simulink model "TST_PIntkVUs_DD"  (R2016b)
settings: Solver=FixedStepDiscrete  StartTime=0.0  StopTime=simTime  FixedStep=sampleTime  RelTol=1e-3
values from neighbouring files (symbols this model uses):
  testCase = 1    [initTST_PIntkVUs_DD_001.m]    (also in initTST_PIntkVUs_DD_002.m = 2; initTST_PIntkVUs_DD_003.m = 3; initTST_PIntkVUs_DD_004.m = 4; initTST_PIntkVUs_DD_005.m = 5)
libraries: UnitTest_Lib x98, simulink x8
(part 1 of 3)
settings Model: Creator=liangyunbo  LastModifiedBy=liangyunbo
settings DebuggingCC: SignalRangeChecking=error

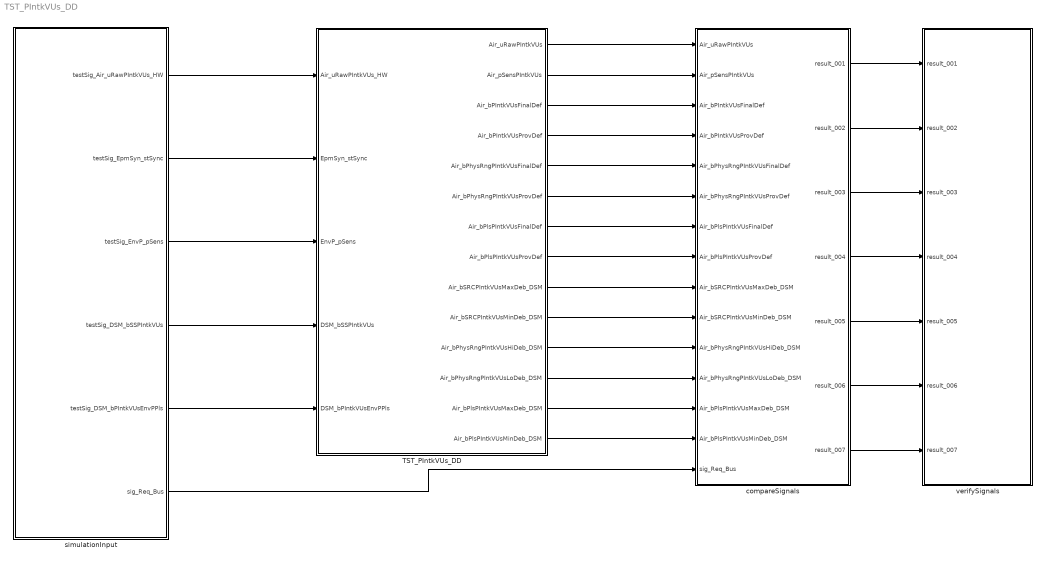
== system TST_PIntkVUs_DD ==
  TST_PIntkVUs_DD : Subsystem
  compareSignals : Subsystem
  simulationInput : Subsystem
  verifySignals : Subsystem
  wires:
  simulationInput/1(testSig_Air_uRawPIntkVUs_HW) -> TST_PIntkVUs_DD/1(Air_uRawPIntkVUs_HW)
  simulationInput/2(testSig_EpmSyn_stSync) -> TST_PIntkVUs_DD/2(EpmSyn_stSync)
  simulationInput/3(testSig_EnvP_pSens) -> TST_PIntkVUs_DD/3(EnvP_pSens)
  simulationInput/4(testSig_DSM_bSSPIntkVUs) -> TST_PIntkVUs_DD/4(DSM_bSSPIntkVUs)
  simulationInput/5(testSig_DSM_bPIntkVUsEnvPPls) -> TST_PIntkVUs_DD/5(DSM_bPIntkVUsEnvPPls)
  TST_PIntkVUs_DD/1(Air_uRawPIntkVUs) -> compareSignals/1(Air_uRawPIntkVUs)
  TST_PIntkVUs_DD/2(Air_pSensPIntkVUs) -> compareSignals/2(Air_pSensPIntkVUs)
  TST_PIntkVUs_DD/3(Air_bPIntkVUsFinalDef) -> compareSignals/3(Air_bPIntkVUsFinalDef)
  TST_PIntkVUs_DD/4(Air_bPIntkVUsProvDef) -> compareSignals/4(Air_bPIntkVUsProvDef)
  TST_PIntkVUs_DD/5(Air_bPhysRngPIntkVUsFinalDef) -> compareSignals/5(Air_bPhysRngPIntkVUsFinalDef)
  TST_PIntkVUs_DD/6(Air_bPhysRngPIntkVUsProvDef) -> compareSignals/6(Air_bPhysRngPIntkVUsProvDef)
  TST_PIntkVUs_DD/7(Air_bPlsPIntkVUsFinalDef) -> compareSignals/7(Air_bPlsPIntkVUsFinalDef)
  TST_PIntkVUs_DD/8(Air_bPlsPIntkVUsProvDef) -> compareSignals/8(Air_bPlsPIntkVUsProvDef)
  TST_PIntkVUs_DD/9(Air_bSRCPIntkVUsMaxDeb_DSM) -> compareSignals/9(Air_bSRCPIntkVUsMaxDeb_DSM)
  TST_PIntkVUs_DD/10(Air_bSRCPIntkVUsMinDeb_DSM) -> compareSignals/10(Air_bSRCPIntkVUsMinDeb_DSM)
  TST_PIntkVUs_DD/11(Air_bPhysRngPIntkVUsHiDeb_DSM) -> compareSignals/11(Air_bPhysRngPIntkVUsHiDeb_DSM)
  TST_PIntkVUs_DD/12(Air_bPhysRngPIntkVUsLoDeb_DSM) -> compareSignals/12(Air_bPhysRngPIntkVUsLoDeb_DSM)
  TST_PIntkVUs_DD/13(Air_bPlsPIntkVUsMaxDeb_DSM) -> compareSignals/13(Air_bPlsPIntkVUsMaxDeb_DSM)
  TST_PIntkVUs_DD/14(Air_bPlsPIntkVUsMinDeb_DSM) -> compareSignals/14(Air_bPlsPIntkVUsMinDeb_DSM)
  simulationInput/6(sig_Req_Bus) -> compareSignals/15(sig_Req_Bus)
  compareSignals/1(result_001) -> verifySignals/1(result_001)
  compareSignals/2(result_002) -> verifySignals/2(result_002)
  compareSignals/3(result_003) -> verifySignals/3(result_003)
  compareSignals/4(result_004) -> verifySignals/4(result_004)
  compareSignals/5(result_005) -> verifySignals/5(result_005)
  compareSignals/6(result_006) -> verifySignals/6(result_006)
  compareSignals/7(result_007) -> verifySignals/7(result_007)

== system TST_PIntkVUs_DD/TST_PIntkVUs_DD ==
  Air_uRawPIntkVUs_HW : Inport
  EpmSyn_stSync : Inport  Port=2
  EnvP_pSens : Inport  Port=3
  DSM_bSSPIntkVUs : Inport  Port=4
  DSM_bPIntkVUsEnvPPls : Inport  Port=5
  Function_Call : simulink/Ports & Subsystems/Function-Call Generator  sample_time=sampleTime  numberOfIterations=1
  PIntkVUs_DD : ModelReference  ModelNameDialog=PIntkVUs_DD  SimulationMode=Normal  ModelReferenceVersion=1.45  TriggerPortName=function  TriggerPortTriggerType=function-call  TriggerPortStatesWhenEnabling=held
  Air_uRawPIntkVUs : Outport
  Air_pSensPIntkVUs : Outport  Port=2
  Air_bPIntkVUsFinalDef : Outport  Port=3
  Air_bPIntkVUsProvDef : Outport  Port=4
  Air_bPhysRngPIntkVUsFinalDef : Outport  Port=5
  Air_bPhysRngPIntkVUsProvDef : Outport  Port=6
  Air_bPlsPIntkVUsFinalDef : Outport  Port=7
  Air_bPlsPIntkVUsProvDef : Outport  Port=8
  Air_bSRCPIntkVUsMaxDeb_DSM : Outport  Port=9
  Air_bSRCPIntkVUsMinDeb_DSM : Outport  Port=10
  Air_bPhysRngPIntkVUsHiDeb_DSM : Outport  Port=11
  Air_bPhysRngPIntkVUsLoDeb_DSM : Outport  Port=12
  Air_bPlsPIntkVUsMaxDeb_DSM : Outport  Port=13
  Air_bPlsPIntkVUsMinDeb_DSM : Outport  Port=14
  wires:
  Function_Call/1 -> PIntkVUs_DD/Trigger
  Air_uRawPIntkVUs_HW/1 -> PIntkVUs_DD/1
  EpmSyn_stSync/1 -> PIntkVUs_DD/2
  EnvP_pSens/1 -> PIntkVUs_DD/3
  DSM_bSSPIntkVUs/1 -> PIntkVUs_DD/4
  DSM_bPIntkVUsEnvPPls/1 -> PIntkVUs_DD/5
  PIntkVUs_DD/1 -> Air_uRawPIntkVUs/1
  PIntkVUs_DD/2 -> Air_pSensPIntkVUs/1
  PIntkVUs_DD/3 -> Air_bPIntkVUsFinalDef/1
  PIntkVUs_DD/4 -> Air_bPIntkVUsProvDef/1
  PIntkVUs_DD/5 -> Air_bPhysRngPIntkVUsFinalDef/1
  PIntkVUs_DD/6 -> Air_bPhysRngPIntkVUsProvDef/1
  PIntkVUs_DD/7 -> Air_bPlsPIntkVUsFinalDef/1
  PIntkVUs_DD/8 -> Air_bPlsPIntkVUsProvDef/1
  PIntkVUs_DD/9 -> Air_bSRCPIntkVUsMaxDeb_DSM/1
  PIntkVUs_DD/10 -> Air_bSRCPIntkVUsMinDeb_DSM/1
  PIntkVUs_DD/11 -> Air_bPhysRngPIntkVUsHiDeb_DSM/1
  PIntkVUs_DD/12 -> Air_bPhysRngPIntkVUsLoDeb_DSM/1
  PIntkVUs_DD/13 -> Air_bPlsPIntkVUsMaxDeb_DSM/1
  PIntkVUs_DD/14 -> Air_bPlsPIntkVUsMinDeb_DSM/1

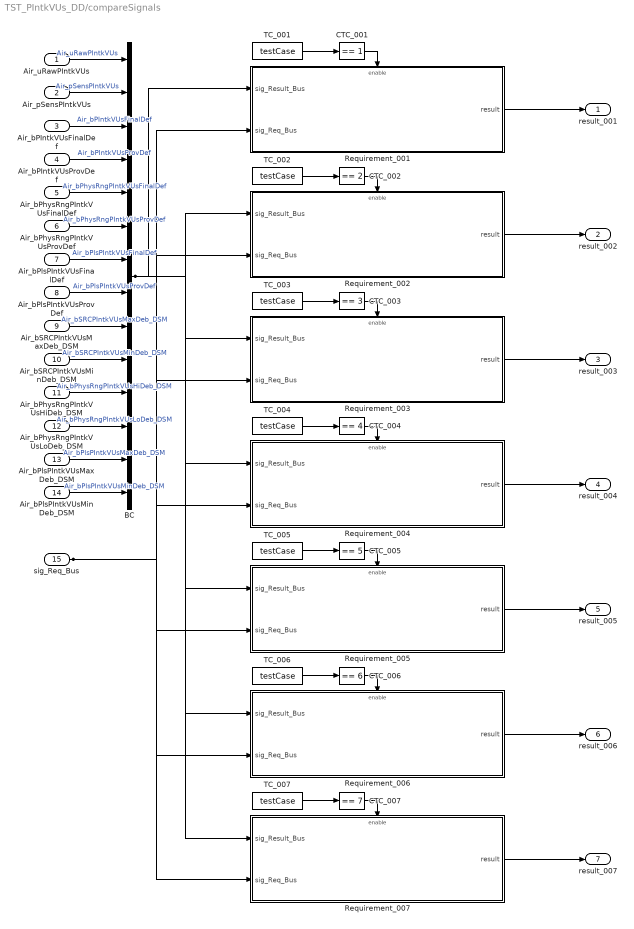
== system TST_PIntkVUs_DD/compareSignals ==
  Air_uRawPIntkVUs : Inport
  Air_pSensPIntkVUs : Inport  Port=2
  Air_bPIntkVUsFinalDef : Inport  Port=3
  Air_bPIntkVUsProvDef : Inport  Port=4
  Air_bPhysRngPIntkVUsFinalDef : Inport  Port=5
  Air_bPhysRngPIntkVUsProvDef : Inport  Port=6
  Air_bPlsPIntkVUsFinalDef : Inport  Port=7
  Air_bPlsPIntkVUsProvDef : Inport  Port=8
  Air_bSRCPIntkVUsMaxDeb_DSM : Inport  Port=9
  Air_bSRCPIntkVUsMinDeb_DSM : Inport  Port=10
  Air_bPhysRngPIntkVUsHiDeb_DSM : Inport  Port=11
  Air_bPhysRngPIntkVUsLoDeb_DSM : Inport  Port=12
  Air_bPlsPIntkVUsMaxDeb_DSM : Inport  Port=13
  Air_bPlsPIntkVUsMinDeb_DSM : Inport  Port=14
  sig_Req_Bus : Inport  Port=15
  BC : BusCreator  Inputs=14
  CTC_001 : simulink/Logic and Bit Operations/Compare To Constant  relop===  const=1  OutDataTypeStr=boolean
  CTC_002 : simulink/Logic and Bit Operations/Compare To Constant  relop===  const=2  OutDataTypeStr=boolean
  CTC_003 : simulink/Logic and Bit Operations/Compare To Constant  relop===  const=3  OutDataTypeStr=boolean
  CTC_004 : simulink/Logic and Bit Operations/Compare To Constant  relop===  const=4  OutDataTypeStr=boolean
  CTC_005 : simulink/Logic and Bit Operations/Compare To Constant  relop===  const=5  OutDataTypeStr=boolean
  CTC_006 : simulink/Logic and Bit Operations/Compare To Constant  relop===  const=6  OutDataTypeStr=boolean
  CTC_007 : simulink/Logic and Bit Operations/Compare To Constant  relop===  const=7  OutDataTypeStr=boolean
  Requirement_001 : Subsystem
  Requirement_002 : Subsystem
  Requirement_003 : Subsystem
  Requirement_004 : Subsystem
  Requirement_005 : Subsystem
  Requirement_006 : Subsystem
  Requirement_007 : Subsystem
  TC_001 : Constant  Value=testCase
  TC_002 : Constant  Value=testCase
  TC_003 : Constant  Value=testCase
  TC_004 : Constant  Value=testCase
  TC_005 : Constant  Value=testCase
  TC_006 : Constant  Value=testCase
  TC_007 : Constant  Value=testCase
  result_001 : Outport
  result_002 : Outport  Port=2
  result_003 : Outport  Port=3
  result_004 : Outport  Port=4
  result_005 : Outport  Port=5
  result_006 : Outport  Port=6
  result_007 : Outport  Port=7
  wires:
  Air_uRawPIntkVUs/1 -> BC/1  "Air_uRawPIntkVUs"
  Air_pSensPIntkVUs/1 -> BC/2  "Air_pSensPIntkVUs"
  Air_bPIntkVUsFinalDef/1 -> BC/3  "Air_bPIntkVUsFinalDef"
  Air_bPIntkVUsProvDef/1 -> BC/4  "Air_bPIntkVUsProvDef"
  Air_bPhysRngPIntkVUsFinalDef/1 -> BC/5  "Air_bPhysRngPIntkVUsFinalDef"
  Air_bPhysRngPIntkVUsProvDef/1 -> BC/6  "Air_bPhysRngPIntkVUsProvDef"
  Air_bPlsPIntkVUsFinalDef/1 -> BC/7  "Air_bPlsPIntkVUsFinalDef"
  Air_bPlsPIntkVUsProvDef/1 -> BC/8  "Air_bPlsPIntkVUsProvDef"
  Air_bSRCPIntkVUsMaxDeb_DSM/1 -> BC/9  "Air_bSRCPIntkVUsMaxDeb_DSM"
  Air_bSRCPIntkVUsMinDeb_DSM/1 -> BC/10  "Air_bSRCPIntkVUsMinDeb_DSM"
  Air_bPhysRngPIntkVUsHiDeb_DSM/1 -> BC/11  "Air_bPhysRngPIntkVUsHiDeb_DSM"
  Air_bPhysRngPIntkVUsLoDeb_DSM/1 -> BC/12  "Air_bPhysRngPIntkVUsLoDeb_DSM"
  Air_bPlsPIntkVUsMaxDeb_DSM/1 -> BC/13  "Air_bPlsPIntkVUsMaxDeb_DSM"
  Air_bPlsPIntkVUsMinDeb_DSM/1 -> BC/14  "Air_bPlsPIntkVUsMinDeb_DSM"
  TC_001/1 -> CTC_001/1
  CTC_001/1 -> Requirement_001/Enable
  sig_Req_Bus/1 -> Requirement_001/2(sig_Req_Bus), Requirement_002/2(sig_Req_Bus), Requirement_003/2(sig_Req_Bus), Requirement_004/2(sig_Req_Bus), Requirement_005/2(sig_Req_Bus), Requirement_006/2(sig_Req_Bus), Requirement_007/2(sig_Req_Bus)
  BC/1 -> Requirement_001/1(sig_Result_Bus), Requirement_002/1(sig_Result_Bus), Requirement_003/1(sig_Result_Bus), Requirement_004/1(sig_Result_Bus), Requirement_005/1(sig_Result_Bus), Requirement_006/1(sig_Result_Bus), Requirement_007/1(sig_Result_Bus)
  Requirement_001/1(result) -> result_001/1
  TC_002/1 -> CTC_002/1
  CTC_002/1 -> Requirement_002/Enable
  Requirement_002/1(result) -> result_002/1
  TC_003/1 -> CTC_003/1
  CTC_003/1 -> Requirement_003/Enable
  Requirement_003/1(result) -> result_003/1
  TC_004/1 -> CTC_004/1
  CTC_004/1 -> Requirement_004/Enable
  Requirement_004/1(result) -> result_004/1
  TC_005/1 -> CTC_005/1
  CTC_005/1 -> Requirement_005/Enable
  Requirement_005/1(result) -> result_005/1
  TC_006/1 -> CTC_006/1
  CTC_006/1 -> Requirement_006/Enable
  Requirement_006/1(result) -> result_006/1
  TC_007/1 -> CTC_007/1
  CTC_007/1 -> Requirement_007/Enable
  Requirement_007/1(result) -> result_007/1

== system TST_PIntkVUs_DD/simulationInput ==
  BS : BusSelector  OutputSignals=testSig_Air_uRawPIntkVUs_HW,testSig_EpmSyn_stSync,testSig_EnvP_pSens,testSig_DSM_bSSPIntkVUs,testSig_DSM_bPIntkVUsEnvPPls
  MPSw : MultiPortSwitch  Inputs=7  SaturateOnIntegerOverflow=on  InputSameDT=on
  TestCase : Constant  Value=testCase
  testSignals_R001 : Subsystem
  testSignals_R002 : Subsystem
  testSignals_R003 : Subsystem
  testSignals_R004 : Subsystem
  testSignals_R005 : Subsystem
  testSignals_R006 : Subsystem
  testSignals_R007 : Subsystem
  testSig_Air_uRawPIntkVUs_HW : Outport
  testSig_EpmSyn_stSync : Outport  Port=2
  testSig_EnvP_pSens : Outport  Port=3
  testSig_DSM_bSSPIntkVUs : Outport  Port=4
  testSig_DSM_bPIntkVUsEnvPPls : Outport  Port=5
  sig_Req_Bus : Outport  Port=6
  wires:
  BS/1 -> testSig_Air_uRawPIntkVUs_HW/1  "<testSig_Air_uRawPIntkVUs_HW>"
  BS/2 -> testSig_EpmSyn_stSync/1  "<testSig_EpmSyn_stSync>"
  BS/3 -> testSig_EnvP_pSens/1  "<testSig_EnvP_pSens>"
  BS/4 -> testSig_DSM_bSSPIntkVUs/1  "<testSig_DSM_bSSPIntkVUs>"
  BS/5 -> testSig_DSM_bPIntkVUsEnvPPls/1  "<testSig_DSM_bPIntkVUsEnvPPls>"
  MPSw/1 -> BS/1, sig_Req_Bus/1
  TestCase/1 -> MPSw/1
  testSignals_R001/1(testSignals) -> MPSw/2
  testSignals_R002/1(testSignals) -> MPSw/3
  testSignals_R003/1(testSignals) -> MPSw/4
  testSignals_R004/1(testSignals) -> MPSw/5
  testSignals_R005/1(testSignals) -> MPSw/6
  testSignals_R006/1(testSignals) -> MPSw/7
  testSignals_R007/1(testSignals) -> MPSw/8

== system TST_PIntkVUs_DD/verifySignals ==
  result_001 : Inport
  result_002 : Inport  Port=2
  result_003 : Inport  Port=3
  result_004 : Inport  Port=4
  result_005 : Inport  Port=5
  result_006 : Inport  Port=6
  result_007 : Inport  Port=7
  Assertion_001 : Assertion  Enabled=off
  Assertion_002 : Assertion  Enabled=off
  Assertion_003 : Assertion  Enabled=off
  Assertion_004 : Assertion  Enabled=off
  Assertion_005 : Assertion  Enabled=off
  Assertion_006 : Assertion  Enabled=off
  Assertion_007 : Assertion  Enabled=off
  wires:
  result_001/1 -> Assertion_001/1
  result_002/1 -> Assertion_002/1
  result_003/1 -> Assertion_003/1
  result_004/1 -> Assertion_004/1
  result_005/1 -> Assertion_005/1
  result_006/1 -> Assertion_006/1
  result_007/1 -> Assertion_007/1

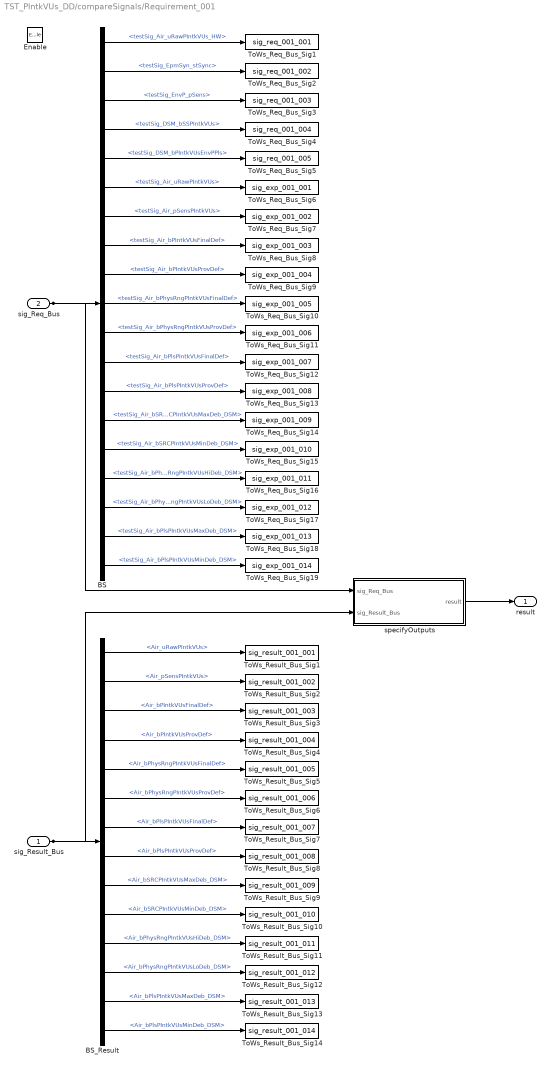
== system TST_PIntkVUs_DD/compareSignals/Requirement_001 ==
  sig_Result_Bus : Inport
  sig_Req_Bus : Inport  Port=2
  Enable : EnablePort
  BS : BusSelector  OutputSignals=testSig_Air_uRawPIntkVUs_HW,testSig_EpmSyn_stSync,testSig_EnvP_pSens,testSig_DSM_bSSPIntkVUs,testSig_DSM_bPIntkVUsEnvPPls,testSig_Air_uRawPIntkVUs,testSig_Air_pSensPIntkVUs,testSig_Air_bPIntkVUsFinalDef,testSig_Air_bPIntkVUsProvDef,testSig_Air_bPhysRngPIntkVUsFinalDef,testSig_Air_bPhysRngPIntkVUsProvDef,testSig_Air_bPlsPIntkVUsFinalDef,testSig_Air_bPlsPIntkVUsProvDef,testSig_Air_bSRCPIntkVUsMaxDeb_DSM,testSig_Air_bSRCPIntkVUsMinDeb_DSM,testSig_Air_bPhysRngPIntkVUsHiDeb_DSM,testSig_Air_bPhysRngPIntkVUsLoDeb_DSM,testSig_Air_bPlsPIntkVUsMaxDeb_DSM,testSig_Air_bPlsPIntkVUsMinDeb_DSM
  BS_Result : BusSelector  OutputSignals=Air_uRawPIntkVUs,Air_pSensPIntkVUs,Air_bPIntkVUsFinalDef,Air_bPIntkVUsProvDef,Air_bPhysRngPIntkVUsFinalDef,Air_bPhysRngPIntkVUsProvDef,Air_bPlsPIntkVUsFinalDef,Air_bPlsPIntkVUsProvDef,Air_bSRCPIntkVUsMaxDeb_DSM,Air_bSRCPIntkVUsMinDeb_DSM,Air_bPhysRngPIntkVUsHiDeb_DSM,Air_bPhysRngPIntkVUsLoDeb_DSM,Air_bPlsPIntkVUsMaxDeb_DSM,Air_bPlsPIntkVUsMinDeb_DSM
  ToWs_Req_Bus_Sig1 : ToWorkspace  VariableName=sig_req_001_001  SaveFormat=Structure With Time
  ToWs_Req_Bus_Sig10 : ToWorkspace  VariableName=sig_exp_001_005  SaveFormat=Structure With Time
  ToWs_Req_Bus_Sig11 : ToWorkspace  VariableName=sig_exp_001_006  SaveFormat=Structure With Time
  ToWs_Req_Bus_Sig12 : ToWorkspace  VariableName=sig_exp_001_007  SaveFormat=Structure With Time
  ToWs_Req_Bus_Sig13 : ToWorkspace  VariableName=sig_exp_001_008  SaveFormat=Structure With Time
  ToWs_Req_Bus_Sig14 : ToWorkspace  VariableName=sig_exp_001_009  SaveFormat=Structure With Time
  ToWs_Req_Bus_Sig15 : ToWorkspace  VariableName=sig_exp_001_010  SaveFormat=Structure With Time
  ToWs_Req_Bus_Sig16 : ToWorkspace  VariableName=sig_exp_001_011  SaveFormat=Structure With Time
  ToWs_Req_Bus_Sig17 : ToWorkspace  VariableName=sig_exp_001_012  SaveFormat=Structure With Time
  ToWs_Req_Bus_Sig18 : ToWorkspace  VariableName=sig_exp_001_013  SaveFormat=Structure With Time
  ToWs_Req_Bus_Sig19 : ToWorkspace  VariableName=sig_exp_001_014  SaveFormat=Structure With Time
  ToWs_Req_Bus_Sig2 : ToWorkspace  VariableName=sig_req_001_002  SaveFormat=Structure With Time
  ToWs_Req_Bus_Sig3 : ToWorkspace  VariableName=sig_req_001_003  SaveFormat=Structure With Time
  ToWs_Req_Bus_Sig4 : ToWorkspace  VariableName=sig_req_001_004  SaveFormat=Structure With Time
  ToWs_Req_Bus_Sig5 : ToWorkspace  VariableName=sig_req_001_005  SaveFormat=Structure With Time
  ToWs_Req_Bus_Sig6 : ToWorkspace  VariableName=sig_exp_001_001  SaveFormat=Structure With Time
  ToWs_Req_Bus_Sig7 : ToWorkspace  VariableName=sig_exp_001_002  SaveFormat=Structure With Time
  ToWs_Req_Bus_Sig8 : ToWorkspace  VariableName=sig_exp_001_003  SaveFormat=Structure With Time
  ToWs_Req_Bus_Sig9 : ToWorkspace  VariableName=sig_exp_001_004  SaveFormat=Structure With Time
  ToWs_Result_Bus_Sig1 : ToWorkspace  VariableName=sig_result_001_001  SaveFormat=Structure With Time
  ToWs_Result_Bus_Sig10 : ToWorkspace  VariableName=sig_result_001_010  SaveFormat=Structure With Time
  ToWs_Result_Bus_Sig11 : ToWorkspace  VariableName=sig_result_001_011  SaveFormat=Structure With Time
  ToWs_Result_Bus_Sig12 : ToWorkspace  VariableName=sig_result_001_012  SaveFormat=Structure With Time
  ToWs_Result_Bus_Sig13 : ToWorkspace  VariableName=sig_result_001_013  SaveFormat=Structure With Time
  ToWs_Result_Bus_Sig14 : ToWorkspace  VariableName=sig_result_001_014  SaveFormat=Structure With Time
  ToWs_Result_Bus_Sig2 : ToWorkspace  VariableName=sig_result_001_002  SaveFormat=Structure With Time
  ToWs_Result_Bus_Sig3 : ToWorkspace  VariableName=sig_result_001_003  SaveFormat=Structure With Time
  ToWs_Result_Bus_Sig4 : ToWorkspace  VariableName=sig_result_001_004  SaveFormat=Structure With Time
  ToWs_Result_Bus_Sig5 : ToWorkspace  VariableName=sig_result_001_005  SaveFormat=Structure With Time
  ToWs_Result_Bus_Sig6 : ToWorkspace  VariableName=sig_result_001_006  SaveFormat=Structure With Time
  ToWs_Result_Bus_Sig7 : ToWorkspace  VariableName=sig_result_001_007  SaveFormat=Structure With Time
  ToWs_Result_Bus_Sig8 : ToWorkspace  VariableName=sig_result_001_008  SaveFormat=Structure With Time
  ToWs_Result_Bus_Sig9 : ToWorkspace  VariableName=sig_result_001_009  SaveFormat=Structure With Time
  specifyOutputs : Subsystem
  result : Outport
  wires:
  sig_Req_Bus/1 -> BS/1, specifyOutputs/1(sig_Req_Bus)
  BS/1 -> ToWs_Req_Bus_Sig1/1  "<testSig_Air_uRawPIntkVUs_HW>"
  BS/2 -> ToWs_Req_Bus_Sig2/1  "<testSig_EpmSyn_stSync>"
  BS/3 -> ToWs_Req_Bus_Sig3/1  "<testSig_EnvP_pSens>"
  BS/4 -> ToWs_Req_Bus_Sig4/1  "<testSig_DSM_bSSPIntkVUs>"
  BS/5 -> ToWs_Req_Bus_Sig5/1  "<testSig_DSM_bPIntkVUsEnvPPls>"
  BS/6 -> ToWs_Req_Bus_Sig6/1  "<testSig_Air_uRawPIntkVUs>"
  BS/7 -> ToWs_Req_Bus_Sig7/1  "<testSig_Air_pSensPIntkVUs>"
  BS/8 -> ToWs_Req_Bus_Sig8/1  "<testSig_Air_bPIntkVUsFinalDef>"
  BS/9 -> ToWs_Req_Bus_Sig9/1  "<testSig_Air_bPIntkVUsProvDef>"
  BS/10 -> ToWs_Req_Bus_Sig10/1  "<testSig_Air_bPhysRngPIntkVUsFinalDef>"
  BS/11 -> ToWs_Req_Bus_Sig11/1  "<testSig_Air_bPhysRngPIntkVUsProvDef>"
  BS/12 -> ToWs_Req_Bus_Sig12/1  "<testSig_Air_bPlsPIntkVUsFinalDef>"
  BS/13 -> ToWs_Req_Bus_Sig13/1  "<testSig_Air_bPlsPIntkVUsProvDef>"
  BS/14 -> ToWs_Req_Bus_Sig14/1  "<testSig_Air_bSRCPIntkVUsMaxDeb_DSM>"
  BS/15 -> ToWs_Req_Bus_Sig15/1  "<testSig_Air_bSRCPIntkVUsMinDeb_DSM>"
  BS/16 -> ToWs_Req_Bus_Sig16/1  "<testSig_Air_bPhysRngPIntkVUsHiDeb_DSM>"
  BS/17 -> ToWs_Req_Bus_Sig17/1  "<testSig_Air_bPhysRngPIntkVUsLoDeb_DSM>"
  BS/18 -> ToWs_Req_Bus_Sig18/1  "<testSig_Air_bPlsPIntkVUsMaxDeb_DSM>"
  BS/19 -> ToWs_Req_Bus_Sig19/1  "<testSig_Air_bPlsPIntkVUsMinDeb_DSM>"
  sig_Result_Bus/1 -> BS_Result/1, specifyOutputs/2(sig_Result_Bus)
  BS_Result/1 -> ToWs_Result_Bus_Sig1/1  "<Air_uRawPIntkVUs>"
  BS_Result/2 -> ToWs_Result_Bus_Sig2/1  "<Air_pSensPIntkVUs>"
  BS_Result/3 -> ToWs_Result_Bus_Sig3/1  "<Air_bPIntkVUsFinalDef>"
  BS_Result/4 -> ToWs_Result_Bus_Sig4/1  "<Air_bPIntkVUsProvDef>"
  BS_Result/5 -> ToWs_Result_Bus_Sig5/1  "<Air_bPhysRngPIntkVUsFinalDef>"
  BS_Result/6 -> ToWs_Result_Bus_Sig6/1  "<Air_bPhysRngPIntkVUsProvDef>"
  BS_Result/7 -> ToWs_Result_Bus_Sig7/1  "<Air_bPlsPIntkVUsFinalDef>"
  BS_Result/8 -> ToWs_Result_Bus_Sig8/1  "<Air_bPlsPIntkVUsProvDef>"
  BS_Result/9 -> ToWs_Result_Bus_Sig9/1  "<Air_bSRCPIntkVUsMaxDeb_DSM>"
  BS_Result/10 -> ToWs_Result_Bus_Sig10/1  "<Air_bSRCPIntkVUsMinDeb_DSM>"
  BS_Result/11 -> ToWs_Result_Bus_Sig11/1  "<Air_bPhysRngPIntkVUsHiDeb_DSM>"
  BS_Result/12 -> ToWs_Result_Bus_Sig12/1  "<Air_bPhysRngPIntkVUsLoDeb_DSM>"
  BS_Result/13 -> ToWs_Result_Bus_Sig13/1  "<Air_bPlsPIntkVUsMaxDeb_DSM>"
  BS_Result/14 -> ToWs_Result_Bus_Sig14/1  "<Air_bPlsPIntkVUsMinDeb_DSM>"
  specifyOutputs/1(result) -> result/1

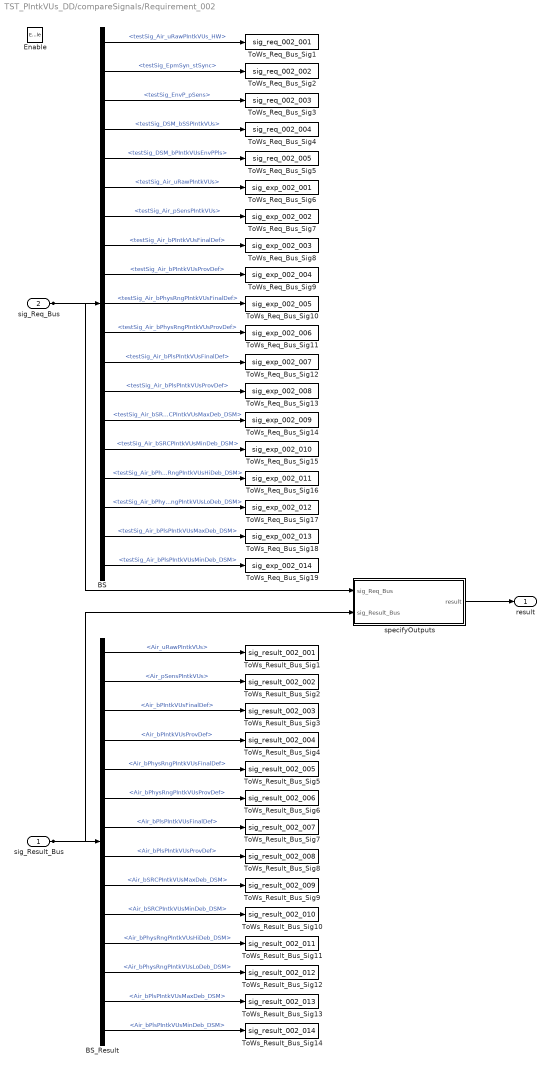
== system TST_PIntkVUs_DD/compareSignals/Requirement_002 ==
  sig_Result_Bus : Inport
  sig_Req_Bus : Inport  Port=2
  Enable : EnablePort
  BS : BusSelector  OutputSignals=testSig_Air_uRawPIntkVUs_HW,testSig_EpmSyn_stSync,testSig_EnvP_pSens,testSig_DSM_bSSPIntkVUs,testSig_DSM_bPIntkVUsEnvPPls,testSig_Air_uRawPIntkVUs,testSig_Air_pSensPIntkVUs,testSig_Air_bPIntkVUsFinalDef,testSig_Air_bPIntkVUsProvDef,testSig_Air_bPhysRngPIntkVUsFinalDef,testSig_Air_bPhysRngPIntkVUsProvDef,testSig_Air_bPlsPIntkVUsFinalDef,testSig_Air_bPlsPIntkVUsProvDef,testSig_Air_bSRCPIntkVUsMaxDeb_DSM,testSig_Air_bSRCPIntkVUsMinDeb_DSM,testSig_Air_bPhysRngPIntkVUsHiDeb_DSM,testSig_Air_bPhysRngPIntkVUsLoDeb_DSM,testSig_Air_bPlsPIntkVUsMaxDeb_DSM,testSig_Air_bPlsPIntkVUsMinDeb_DSM
  BS_Result : BusSelector  OutputSignals=Air_uRawPIntkVUs,Air_pSensPIntkVUs,Air_bPIntkVUsFinalDef,Air_bPIntkVUsProvDef,Air_bPhysRngPIntkVUsFinalDef,Air_bPhysRngPIntkVUsProvDef,Air_bPlsPIntkVUsFinalDef,Air_bPlsPIntkVUsProvDef,Air_bSRCPIntkVUsMaxDeb_DSM,Air_bSRCPIntkVUsMinDeb_DSM,Air_bPhysRngPIntkVUsHiDeb_DSM,Air_bPhysRngPIntkVUsLoDeb_DSM,Air_bPlsPIntkVUsMaxDeb_DSM,Air_bPlsPIntkVUsMinDeb_DSM
  ToWs_Req_Bus_Sig1 : ToWorkspace  VariableName=sig_req_002_001  SaveFormat=Structure With Time
  ToWs_Req_Bus_Sig10 : ToWorkspace  VariableName=sig_exp_002_005  SaveFormat=Structure With Time
  ToWs_Req_Bus_Sig11 : ToWorkspace  VariableName=sig_exp_002_006  SaveFormat=Structure With Time
  ToWs_Req_Bus_Sig12 : ToWorkspace  VariableName=sig_exp_002_007  SaveFormat=Structure With Time
  ToWs_Req_Bus_Sig13 : ToWorkspace  VariableName=sig_exp_002_008  SaveFormat=Structure With Time
  ToWs_Req_Bus_Sig14 : ToWorkspace  VariableName=sig_exp_002_009  SaveFormat=Structure With Time
  ToWs_Req_Bus_Sig15 : ToWorkspace  VariableName=sig_exp_002_010  SaveFormat=Structure With Time
  ToWs_Req_Bus_Sig16 : ToWorkspace  VariableName=sig_exp_002_011  SaveFormat=Structure With Time
  ToWs_Req_Bus_Sig17 : ToWorkspace  VariableName=sig_exp_002_012  SaveFormat=Structure With Time
  ToWs_Req_Bus_Sig18 : ToWorkspace  VariableName=sig_exp_002_013  SaveFormat=Structure With Time
  ToWs_Req_Bus_Sig19 : ToWorkspace  VariableName=sig_exp_002_014  SaveFormat=Structure With Time
  ToWs_Req_Bus_Sig2 : ToWorkspace  VariableName=sig_req_002_002  SaveFormat=Structure With Time
  ToWs_Req_Bus_Sig3 : ToWorkspace  VariableName=sig_req_002_003  SaveFormat=Structure With Time
  ToWs_Req_Bus_Sig4 : ToWorkspace  VariableName=sig_req_002_004  SaveFormat=Structure With Time
  ToWs_Req_Bus_Sig5 : ToWorkspace  VariableName=sig_req_002_005  SaveFormat=Structure With Time
  ToWs_Req_Bus_Sig6 : ToWorkspace  VariableName=sig_exp_002_001  SaveFormat=Structure With Time
  ToWs_Req_Bus_Sig7 : ToWorkspace  VariableName=sig_exp_002_002  SaveFormat=Structure With Time
  ToWs_Req_Bus_Sig8 : ToWorkspace  VariableName=sig_exp_002_003  SaveFormat=Structure With Time
  ToWs_Req_Bus_Sig9 : ToWorkspace  VariableName=sig_exp_002_004  SaveFormat=Structure With Time
  ToWs_Result_Bus_Sig1 : ToWorkspace  VariableName=sig_result_002_001  SaveFormat=Structure With Time
  ToWs_Result_Bus_Sig10 : ToWorkspace  VariableName=sig_result_002_010  SaveFormat=Structure With Time
  ToWs_Result_Bus_Sig11 : ToWorkspace  VariableName=sig_result_002_011  SaveFormat=Structure With Time
  ToWs_Result_Bus_Sig12 : ToWorkspace  VariableName=sig_result_002_012  SaveFormat=Structure With Time
  ToWs_Result_Bus_Sig13 : ToWorkspace  VariableName=sig_result_002_013  SaveFormat=Structure With Time
  ToWs_Result_Bus_Sig14 : ToWorkspace  VariableName=sig_result_002_014  SaveFormat=Structure With Time
  ToWs_Result_Bus_Sig2 : ToWorkspace  VariableName=sig_result_002_002  SaveFormat=Structure With Time
  ToWs_Result_Bus_Sig3 : ToWorkspace  VariableName=sig_result_002_003  SaveFormat=Structure With Time
  ToWs_Result_Bus_Sig4 : ToWorkspace  VariableName=sig_result_002_004  SaveFormat=Structure With Time
  ToWs_Result_Bus_Sig5 : ToWorkspace  VariableName=sig_result_002_005  SaveFormat=Structure With Time
  ToWs_Result_Bus_Sig6 : ToWorkspace  VariableName=sig_result_002_006  SaveFormat=Structure With Time
  ToWs_Result_Bus_Sig7 : ToWorkspace  VariableName=sig_result_002_007  SaveFormat=Structure With Time
  ToWs_Result_Bus_Sig8 : ToWorkspace  VariableName=sig_result_002_008  SaveFormat=Structure With Time
  ToWs_Result_Bus_Sig9 : ToWorkspace  VariableName=sig_result_002_009  SaveFormat=Structure With Time
  specifyOutputs : Subsystem
  result : Outport
  wires:
  sig_Req_Bus/1 -> BS/1, specifyOutputs/1(sig_Req_Bus)
  BS/1 -> ToWs_Req_Bus_Sig1/1  "<testSig_Air_uRawPIntkVUs_HW>"
  BS/2 -> ToWs_Req_Bus_Sig2/1  "<testSig_EpmSyn_stSync>"
  BS/3 -> ToWs_Req_Bus_Sig3/1  "<testSig_EnvP_pSens>"
  BS/4 -> ToWs_Req_Bus_Sig4/1  "<testSig_DSM_bSSPIntkVUs>"
  BS/5 -> ToWs_Req_Bus_Sig5/1  "<testSig_DSM_bPIntkVUsEnvPPls>"
  BS/6 -> ToWs_Req_Bus_Sig6/1  "<testSig_Air_uRawPIntkVUs>"
  BS/7 -> ToWs_Req_Bus_Sig7/1  "<testSig_Air_pSensPIntkVUs>"
  BS/8 -> ToWs_Req_Bus_Sig8/1  "<testSig_Air_bPIntkVUsFinalDef>"
  BS/9 -> ToWs_Req_Bus_Sig9/1  "<testSig_Air_bPIntkVUsProvDef>"
  BS/10 -> ToWs_Req_Bus_Sig10/1  "<testSig_Air_bPhysRngPIntkVUsFinalDef>"
  BS/11 -> ToWs_Req_Bus_Sig11/1  "<testSig_Air_bPhysRngPIntkVUsProvDef>"
  BS/12 -> ToWs_Req_Bus_Sig12/1  "<testSig_Air_bPlsPIntkVUsFinalDef>"
  BS/13 -> ToWs_Req_Bus_Sig13/1  "<testSig_Air_bPlsPIntkVUsProvDef>"
  BS/14 -> ToWs_Req_Bus_Sig14/1  "<testSig_Air_bSRCPIntkVUsMaxDeb_DSM>"
  BS/15 -> ToWs_Req_Bus_Sig15/1  "<testSig_Air_bSRCPIntkVUsMinDeb_DSM>"
  BS/16 -> ToWs_Req_Bus_Sig16/1  "<testSig_Air_bPhysRngPIntkVUsHiDeb_DSM>"
  BS/17 -> ToWs_Req_Bus_Sig17/1  "<testSig_Air_bPhysRngPIntkVUsLoDeb_DSM>"
  BS/18 -> ToWs_Req_Bus_Sig18/1  "<testSig_Air_bPlsPIntkVUsMaxDeb_DSM>"
  BS/19 -> ToWs_Req_Bus_Sig19/1  "<testSig_Air_bPlsPIntkVUsMinDeb_DSM>"
  sig_Result_Bus/1 -> BS_Result/1, specifyOutputs/2(sig_Result_Bus)
  BS_Result/1 -> ToWs_Result_Bus_Sig1/1  "<Air_uRawPIntkVUs>"
  BS_Result/2 -> ToWs_Result_Bus_Sig2/1  "<Air_pSensPIntkVUs>"
  BS_Result/3 -> ToWs_Result_Bus_Sig3/1  "<Air_bPIntkVUsFinalDef>"
  BS_Result/4 -> ToWs_Result_Bus_Sig4/1  "<Air_bPIntkVUsProvDef>"
  BS_Result/5 -> ToWs_Result_Bus_Sig5/1  "<Air_bPhysRngPIntkVUsFinalDef>"
  BS_Result/6 -> ToWs_Result_Bus_Sig6/1  "<Air_bPhysRngPIntkVUsProvDef>"
  BS_Result/7 -> ToWs_Result_Bus_Sig7/1  "<Air_bPlsPIntkVUsFinalDef>"
  BS_Result/8 -> ToWs_Result_Bus_Sig8/1  "<Air_bPlsPIntkVUsProvDef>"
  BS_Result/9 -> ToWs_Result_Bus_Sig9/1  "<Air_bSRCPIntkVUsMaxDeb_DSM>"
  BS_Result/10 -> ToWs_Result_Bus_Sig10/1  "<Air_bSRCPIntkVUsMinDeb_DSM>"
  BS_Result/11 -> ToWs_Result_Bus_Sig11/1  "<Air_bPhysRngPIntkVUsHiDeb_DSM>"
  BS_Result/12 -> ToWs_Result_Bus_Sig12/1  "<Air_bPhysRngPIntkVUsLoDeb_DSM>"
  BS_Result/13 -> ToWs_Result_Bus_Sig13/1  "<Air_bPlsPIntkVUsMaxDeb_DSM>"
  BS_Result/14 -> ToWs_Result_Bus_Sig14/1  "<Air_bPlsPIntkVUsMinDeb_DSM>"
  specifyOutputs/1(result) -> result/1

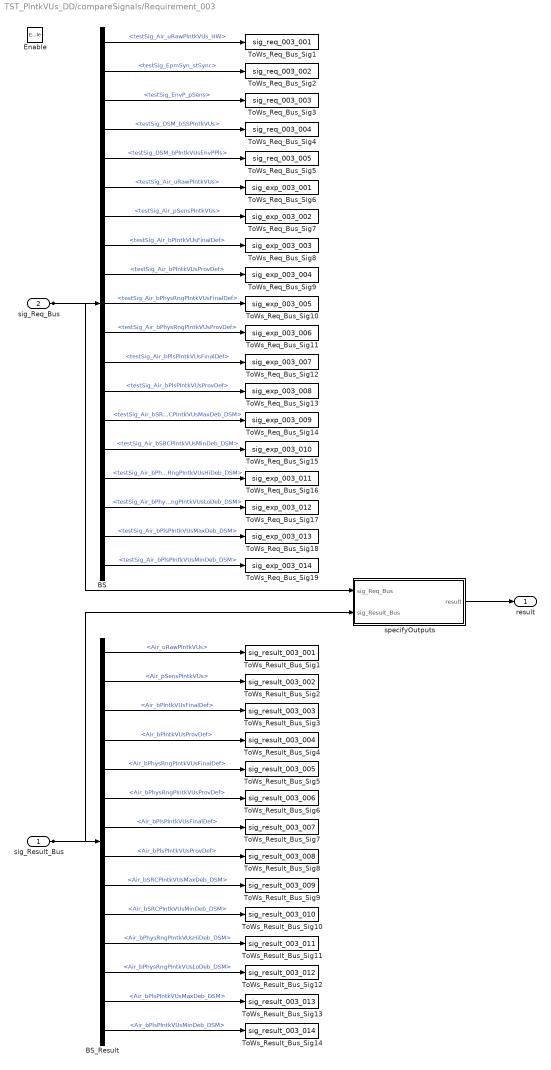
== system TST_PIntkVUs_DD/compareSignals/Requirement_003 ==
  sig_Result_Bus : Inport
  sig_Req_Bus : Inport  Port=2
  Enable : EnablePort
  BS : BusSelector  OutputSignals=testSig_Air_uRawPIntkVUs_HW,testSig_EpmSyn_stSync,testSig_EnvP_pSens,testSig_DSM_bSSPIntkVUs,testSig_DSM_bPIntkVUsEnvPPls,testSig_Air_uRawPIntkVUs,testSig_Air_pSensPIntkVUs,testSig_Air_bPIntkVUsFinalDef,testSig_Air_bPIntkVUsProvDef,testSig_Air_bPhysRngPIntkVUsFinalDef,testSig_Air_bPhysRngPIntkVUsProvDef,testSig_Air_bPlsPIntkVUsFinalDef,testSig_Air_bPlsPIntkVUsProvDef,testSig_Air_bSRCPIntkVUsMaxDeb_DSM,testSig_Air_bSRCPIntkVUsMinDeb_DSM,testSig_Air_bPhysRngPIntkVUsHiDeb_DSM,testSig_Air_bPhysRngPIntkVUsLoDeb_DSM,testSig_Air_bPlsPIntkVUsMaxDeb_DSM,testSig_Air_bPlsPIntkVUsMinDeb_DSM
  BS_Result : BusSelector  OutputSignals=Air_uRawPIntkVUs,Air_pSensPIntkVUs,Air_bPIntkVUsFinalDef,Air_bPIntkVUsProvDef,Air_bPhysRngPIntkVUsFinalDef,Air_bPhysRngPIntkVUsProvDef,Air_bPlsPIntkVUsFinalDef,Air_bPlsPIntkVUsProvDef,Air_bSRCPIntkVUsMaxDeb_DSM,Air_bSRCPIntkVUsMinDeb_DSM,Air_bPhysRngPIntkVUsHiDeb_DSM,Air_bPhysRngPIntkVUsLoDeb_DSM,Air_bPlsPIntkVUsMaxDeb_DSM,Air_bPlsPIntkVUsMinDeb_DSM
  ToWs_Req_Bus_Sig1 : ToWorkspace  VariableName=sig_req_003_001  SaveFormat=Structure With Time
  ToWs_Req_Bus_Sig10 : ToWorkspace  VariableName=sig_exp_003_005  SaveFormat=Structure With Time
  ToWs_Req_Bus_Sig11 : ToWorkspace  VariableName=sig_exp_003_006  SaveFormat=Structure With Time
  ToWs_Req_Bus_Sig12 : ToWorkspace  VariableName=sig_exp_003_007  SaveFormat=Structure With Time
  ToWs_Req_Bus_Sig13 : ToWorkspace  VariableName=sig_exp_003_008  SaveFormat=Structure With Time
  ToWs_Req_Bus_Sig14 : ToWorkspace  VariableName=sig_exp_003_009  SaveFormat=Structure With Time
  ToWs_Req_Bus_Sig15 : ToWorkspace  VariableName=sig_exp_003_010  SaveFormat=Structure With Time
  ToWs_Req_Bus_Sig16 : ToWorkspace  VariableName=sig_exp_003_011  SaveFormat=Structure With Time
  ToWs_Req_Bus_Sig17 : ToWorkspace  VariableName=sig_exp_003_012  SaveFormat=Structure With Time
  ToWs_Req_Bus_Sig18 : ToWorkspace  VariableName=sig_exp_003_013  SaveFormat=Structure With Time
  ToWs_Req_Bus_Sig19 : ToWorkspace  VariableName=sig_exp_003_014  SaveFormat=Structure With Time
  ToWs_Req_Bus_Sig2 : ToWorkspace  VariableName=sig_req_003_002  SaveFormat=Structure With Time
  ToWs_Req_Bus_Sig3 : ToWorkspace  VariableName=sig_req_003_003  SaveFormat=Structure With Time
  ToWs_Req_Bus_Sig4 : ToWorkspace  VariableName=sig_req_003_004  SaveFormat=Structure With Time
  ToWs_Req_Bus_Sig5 : ToWorkspace  VariableName=sig_req_003_005  SaveFormat=Structure With Time
  ToWs_Req_Bus_Sig6 : ToWorkspace  VariableName=sig_exp_003_001  SaveFormat=Structure With Time
  ToWs_Req_Bus_Sig7 : ToWorkspace  VariableName=sig_exp_003_002  SaveFormat=Structure With Time
  ToWs_Req_Bus_Sig8 : ToWorkspace  VariableName=sig_exp_003_003  SaveFormat=Structure With Time
  ToWs_Req_Bus_Sig9 : ToWorkspace  VariableName=sig_exp_003_004  SaveFormat=Structure With Time
  ToWs_Result_Bus_Sig1 : ToWorkspace  VariableName=sig_result_003_001  SaveFormat=Structure With Time
  ToWs_Result_Bus_Sig10 : ToWorkspace  VariableName=sig_result_003_010  SaveFormat=Structure With Time
  ToWs_Result_Bus_Sig11 : ToWorkspace  VariableName=sig_result_003_011  SaveFormat=Structure With Time
  ToWs_Result_Bus_Sig12 : ToWorkspace  VariableName=sig_result_003_012  SaveFormat=Structure With Time
  ToWs_Result_Bus_Sig13 : ToWorkspace  VariableName=sig_result_003_013  SaveFormat=Structure With Time
  ToWs_Result_Bus_Sig14 : ToWorkspace  VariableName=sig_result_003_014  SaveFormat=Structure With Time
  ToWs_Result_Bus_Sig2 : ToWorkspace  VariableName=sig_result_003_002  SaveFormat=Structure With Time
  ToWs_Result_Bus_Sig3 : ToWorkspace  VariableName=sig_result_003_003  SaveFormat=Structure With Time
  ToWs_Result_Bus_Sig4 : ToWorkspace  VariableName=sig_result_003_004  SaveFormat=Structure With Time
  ToWs_Result_Bus_Sig5 : ToWorkspace  VariableName=sig_result_003_005  SaveFormat=Structure With Time
  ToWs_Result_Bus_Sig6 : ToWorkspace  VariableName=sig_result_003_006  SaveFormat=Structure With Time
  ToWs_Result_Bus_Sig7 : ToWorkspace  VariableName=sig_result_003_007  SaveFormat=Structure With Time
  ToWs_Result_Bus_Sig8 : ToWorkspace  VariableName=sig_result_003_008  SaveFormat=Structure With Time
  ToWs_Result_Bus_Sig9 : ToWorkspace  VariableName=sig_result_003_009  SaveFormat=Structure With Time
  specifyOutputs : Subsystem
  result : Outport
  wires:
  sig_Req_Bus/1 -> BS/1, specifyOutputs/1(sig_Req_Bus)
  BS/1 -> ToWs_Req_Bus_Sig1/1  "<testSig_Air_uRawPIntkVUs_HW>"
  BS/2 -> ToWs_Req_Bus_Sig2/1  "<testSig_EpmSyn_stSync>"
  BS/3 -> ToWs_Req_Bus_Sig3/1  "<testSig_EnvP_pSens>"
  BS/4 -> ToWs_Req_Bus_Sig4/1  "<testSig_DSM_bSSPIntkVUs>"
  BS/5 -> ToWs_Req_Bus_Sig5/1  "<testSig_DSM_bPIntkVUsEnvPPls>"
  BS/6 -> ToWs_Req_Bus_Sig6/1  "<testSig_Air_uRawPIntkVUs>"
  BS/7 -> ToWs_Req_Bus_Sig7/1  "<testSig_Air_pSensPIntkVUs>"
  BS/8 -> ToWs_Req_Bus_Sig8/1  "<testSig_Air_bPIntkVUsFinalDef>"
  BS/9 -> ToWs_Req_Bus_Sig9/1  "<testSig_Air_bPIntkVUsProvDef>"
  BS/10 -> ToWs_Req_Bus_Sig10/1  "<testSig_Air_bPhysRngPIntkVUsFinalDef>"
  BS/11 -> ToWs_Req_Bus_Sig11/1  "<testSig_Air_bPhysRngPIntkVUsProvDef>"
  BS/12 -> ToWs_Req_Bus_Sig12/1  "<testSig_Air_bPlsPIntkVUsFinalDef>"
  BS/13 -> ToWs_Req_Bus_Sig13/1  "<testSig_Air_bPlsPIntkVUsProvDef>"
  BS/14 -> ToWs_Req_Bus_Sig14/1  "<testSig_Air_bSRCPIntkVUsMaxDeb_DSM>"
  BS/15 -> ToWs_Req_Bus_Sig15/1  "<testSig_Air_bSRCPIntkVUsMinDeb_DSM>"
  BS/16 -> ToWs_Req_Bus_Sig16/1  "<testSig_Air_bPhysRngPIntkVUsHiDeb_DSM>"
  BS/17 -> ToWs_Req_Bus_Sig17/1  "<testSig_Air_bPhysRngPIntkVUsLoDeb_DSM>"
  BS/18 -> ToWs_Req_Bus_Sig18/1  "<testSig_Air_bPlsPIntkVUsMaxDeb_DSM>"
  BS/19 -> ToWs_Req_Bus_Sig19/1  "<testSig_Air_bPlsPIntkVUsMinDeb_DSM>"
  sig_Result_Bus/1 -> BS_Result/1, specifyOutputs/2(sig_Result_Bus)
  BS_Result/1 -> ToWs_Result_Bus_Sig1/1  "<Air_uRawPIntkVUs>"
  BS_Result/2 -> ToWs_Result_Bus_Sig2/1  "<Air_pSensPIntkVUs>"
  BS_Result/3 -> ToWs_Result_Bus_Sig3/1  "<Air_bPIntkVUsFinalDef>"
  BS_Result/4 -> ToWs_Result_Bus_Sig4/1  "<Air_bPIntkVUsProvDef>"
  BS_Result/5 -> ToWs_Result_Bus_Sig5/1  "<Air_bPhysRngPIntkVUsFinalDef>"
  BS_Result/6 -> ToWs_Result_Bus_Sig6/1  "<Air_bPhysRngPIntkVUsProvDef>"
  BS_Result/7 -> ToWs_Result_Bus_Sig7/1  "<Air_bPlsPIntkVUsFinalDef>"
  BS_Result/8 -> ToWs_Result_Bus_Sig8/1  "<Air_bPlsPIntkVUsProvDef>"
  BS_Result/9 -> ToWs_Result_Bus_Sig9/1  "<Air_bSRCPIntkVUsMaxDeb_DSM>"
  BS_Result/10 -> ToWs_Result_Bus_Sig10/1  "<Air_bSRCPIntkVUsMinDeb_DSM>"
  BS_Result/11 -> ToWs_Result_Bus_Sig11/1  "<Air_bPhysRngPIntkVUsHiDeb_DSM>"
  BS_Result/12 -> ToWs_Result_Bus_Sig12/1  "<Air_bPhysRngPIntkVUsLoDeb_DSM>"
  BS_Result/13 -> ToWs_Result_Bus_Sig13/1  "<Air_bPlsPIntkVUsMaxDeb_DSM>"
  BS_Result/14 -> ToWs_Result_Bus_Sig14/1  "<Air_bPlsPIntkVUsMinDeb_DSM>"
  specifyOutputs/1(result) -> result/1

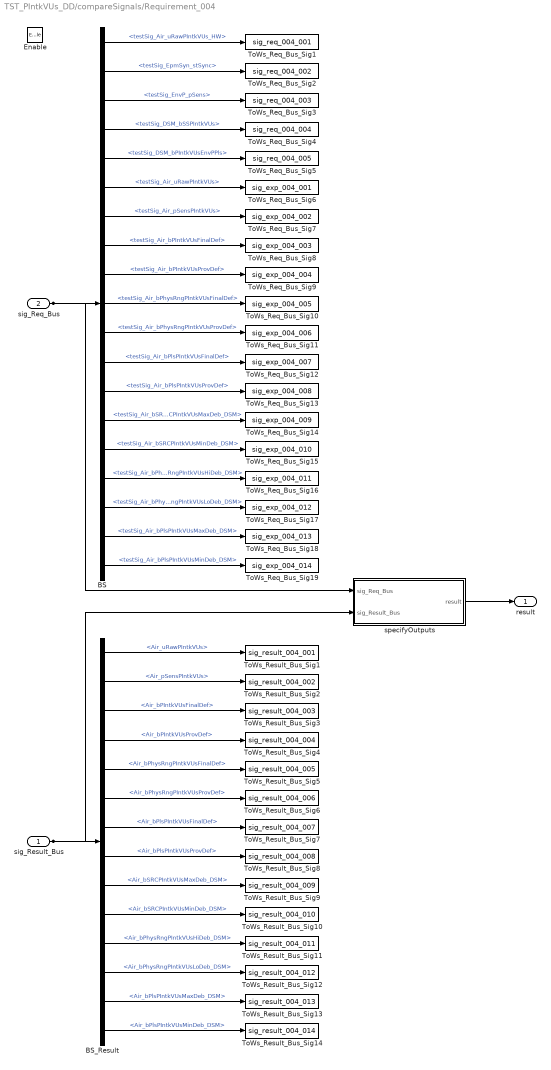
== system TST_PIntkVUs_DD/compareSignals/Requirement_004 ==
  sig_Result_Bus : Inport
  sig_Req_Bus : Inport  Port=2
  Enable : EnablePort
  BS : BusSelector  OutputSignals=testSig_Air_uRawPIntkVUs_HW,testSig_EpmSyn_stSync,testSig_EnvP_pSens,testSig_DSM_bSSPIntkVUs,testSig_DSM_bPIntkVUsEnvPPls,testSig_Air_uRawPIntkVUs,testSig_Air_pSensPIntkVUs,testSig_Air_bPIntkVUsFinalDef,testSig_Air_bPIntkVUsProvDef,testSig_Air_bPhysRngPIntkVUsFinalDef,testSig_Air_bPhysRngPIntkVUsProvDef,testSig_Air_bPlsPIntkVUsFinalDef,testSig_Air_bPlsPIntkVUsProvDef,testSig_Air_bSRCPIntkVUsMaxDeb_DSM,testSig_Air_bSRCPIntkVUsMinDeb_DSM,testSig_Air_bPhysRngPIntkVUsHiDeb_DSM,testSig_Air_bPhysRngPIntkVUsLoDeb_DSM,testSig_Air_bPlsPIntkVUsMaxDeb_DSM,testSig_Air_bPlsPIntkVUsMinDeb_DSM
  BS_Result : BusSelector  OutputSignals=Air_uRawPIntkVUs,Air_pSensPIntkVUs,Air_bPIntkVUsFinalDef,Air_bPIntkVUsProvDef,Air_bPhysRngPIntkVUsFinalDef,Air_bPhysRngPIntkVUsProvDef,Air_bPlsPIntkVUsFinalDef,Air_bPlsPIntkVUsProvDef,Air_bSRCPIntkVUsMaxDeb_DSM,Air_bSRCPIntkVUsMinDeb_DSM,Air_bPhysRngPIntkVUsHiDeb_DSM,Air_bPhysRngPIntkVUsLoDeb_DSM,Air_bPlsPIntkVUsMaxDeb_DSM,Air_bPlsPIntkVUsMinDeb_DSM
  ToWs_Req_Bus_Sig1 : ToWorkspace  VariableName=sig_req_004_001  SaveFormat=Structure With Time
  ToWs_Req_Bus_Sig10 : ToWorkspace  VariableName=sig_exp_004_005  SaveFormat=Structure With Time
  ToWs_Req_Bus_Sig11 : ToWorkspace  VariableName=sig_exp_004_006  SaveFormat=Structure With Time
  ToWs_Req_Bus_Sig12 : ToWorkspace  VariableName=sig_exp_004_007  SaveFormat=Structure With Time
  ToWs_Req_Bus_Sig13 : ToWorkspace  VariableName=sig_exp_004_008  SaveFormat=Structure With Time
  ToWs_Req_Bus_Sig14 : ToWorkspace  VariableName=sig_exp_004_009  SaveFormat=Structure With Time
  ToWs_Req_Bus_Sig15 : ToWorkspace  VariableName=sig_exp_004_010  SaveFormat=Structure With Time
  ToWs_Req_Bus_Sig16 : ToWorkspace  VariableName=sig_exp_004_011  SaveFormat=Structure With Time
  ToWs_Req_Bus_Sig17 : ToWorkspace  VariableName=sig_exp_004_012  SaveFormat=Structure With Time
  ToWs_Req_Bus_Sig18 : ToWorkspace  VariableName=sig_exp_004_013  SaveFormat=Structure With Time
  ToWs_Req_Bus_Sig19 : ToWorkspace  VariableName=sig_exp_004_014  SaveFormat=Structure With Time
  ToWs_Req_Bus_Sig2 : ToWorkspace  VariableName=sig_req_004_002  SaveFormat=Structure With Time
  ToWs_Req_Bus_Sig3 : ToWorkspace  VariableName=sig_req_004_003  SaveFormat=Structure With Time
  ToWs_Req_Bus_Sig4 : ToWorkspace  VariableName=sig_req_004_004  SaveFormat=Structure With Time
  ToWs_Req_Bus_Sig5 : ToWorkspace  VariableName=sig_req_004_005  SaveFormat=Structure With Time
  ToWs_Req_Bus_Sig6 : ToWorkspace  VariableName=sig_exp_004_001  SaveFormat=Structure With Time
  ToWs_Req_Bus_Sig7 : ToWorkspace  VariableName=sig_exp_004_002  SaveFormat=Structure With Time
  ToWs_Req_Bus_Sig8 : ToWorkspace  VariableName=sig_exp_004_003  SaveFormat=Structure With Time
  ToWs_Req_Bus_Sig9 : ToWorkspace  VariableName=sig_exp_004_004  SaveFormat=Structure With Time
  ToWs_Result_Bus_Sig1 : ToWorkspace  VariableName=sig_result_004_001  SaveFormat=Structure With Time
  ToWs_Result_Bus_Sig10 : ToWorkspace  VariableName=sig_result_004_010  SaveFormat=Structure With Time
  ToWs_Result_Bus_Sig11 : ToWorkspace  VariableName=sig_result_004_011  SaveFormat=Structure With Time
  ToWs_Result_Bus_Sig12 : ToWorkspace  VariableName=sig_result_004_012  SaveFormat=Structure With Time
  ToWs_Result_Bus_Sig13 : ToWorkspace  VariableName=sig_result_004_013  SaveFormat=Structure With Time
  ToWs_Result_Bus_Sig14 : ToWorkspace  VariableName=sig_result_004_014  SaveFormat=Structure With Time
  ToWs_Result_Bus_Sig2 : ToWorkspace  VariableName=sig_result_004_002  SaveFormat=Structure With Time
  ToWs_Result_Bus_Sig3 : ToWorkspace  VariableName=sig_result_004_003  SaveFormat=Structure With Time
  ToWs_Result_Bus_Sig4 : ToWorkspace  VariableName=sig_result_004_004  SaveFormat=Structure With Time
  ToWs_Result_Bus_Sig5 : ToWorkspace  VariableName=sig_result_004_005  SaveFormat=Structure With Time
  ToWs_Result_Bus_Sig6 : ToWorkspace  VariableName=sig_result_004_006  SaveFormat=Structure With Time
  ToWs_Result_Bus_Sig7 : ToWorkspace  VariableName=sig_result_004_007  SaveFormat=Structure With Time
  ToWs_Result_Bus_Sig8 : ToWorkspace  VariableName=sig_result_004_008  SaveFormat=Structure With Time
  ToWs_Result_Bus_Sig9 : ToWorkspace  VariableName=sig_result_004_009  SaveFormat=Structure With Time
  specifyOutputs : Subsystem
  result : Outport
  wires:
  sig_Req_Bus/1 -> BS/1, specifyOutputs/1(sig_Req_Bus)
  BS/1 -> ToWs_Req_Bus_Sig1/1  "<testSig_Air_uRawPIntkVUs_HW>"
  BS/2 -> ToWs_Req_Bus_Sig2/1  "<testSig_EpmSyn_stSync>"
  BS/3 -> ToWs_Req_Bus_Sig3/1  "<testSig_EnvP_pSens>"
  BS/4 -> ToWs_Req_Bus_Sig4/1  "<testSig_DSM_bSSPIntkVUs>"
  BS/5 -> ToWs_Req_Bus_Sig5/1  "<testSig_DSM_bPIntkVUsEnvPPls>"
  BS/6 -> ToWs_Req_Bus_Sig6/1  "<testSig_Air_uRawPIntkVUs>"
  BS/7 -> ToWs_Req_Bus_Sig7/1  "<testSig_Air_pSensPIntkVUs>"
  BS/8 -> ToWs_Req_Bus_Sig8/1  "<testSig_Air_bPIntkVUsFinalDef>"
  BS/9 -> ToWs_Req_Bus_Sig9/1  "<testSig_Air_bPIntkVUsProvDef>"
  BS/10 -> ToWs_Req_Bus_Sig10/1  "<testSig_Air_bPhysRngPIntkVUsFinalDef>"
  BS/11 -> ToWs_Req_Bus_Sig11/1  "<testSig_Air_bPhysRngPIntkVUsProvDef>"
  BS/12 -> ToWs_Req_Bus_Sig12/1  "<testSig_Air_bPlsPIntkVUsFinalDef>"
  BS/13 -> ToWs_Req_Bus_Sig13/1  "<testSig_Air_bPlsPIntkVUsProvDef>"
  BS/14 -> ToWs_Req_Bus_Sig14/1  "<testSig_Air_bSRCPIntkVUsMaxDeb_DSM>"
  BS/15 -> ToWs_Req_Bus_Sig15/1  "<testSig_Air_bSRCPIntkVUsMinDeb_DSM>"
  BS/16 -> ToWs_Req_Bus_Sig16/1  "<testSig_Air_bPhysRngPIntkVUsHiDeb_DSM>"
  BS/17 -> ToWs_Req_Bus_Sig17/1  "<testSig_Air_bPhysRngPIntkVUsLoDeb_DSM>"
  BS/18 -> ToWs_Req_Bus_Sig18/1  "<testSig_Air_bPlsPIntkVUsMaxDeb_DSM>"
  BS/19 -> ToWs_Req_Bus_Sig19/1  "<testSig_Air_bPlsPIntkVUsMinDeb_DSM>"
  sig_Result_Bus/1 -> BS_Result/1, specifyOutputs/2(sig_Result_Bus)
  BS_Result/1 -> ToWs_Result_Bus_Sig1/1  "<Air_uRawPIntkVUs>"
  BS_Result/2 -> ToWs_Result_Bus_Sig2/1  "<Air_pSensPIntkVUs>"
  BS_Result/3 -> ToWs_Result_Bus_Sig3/1  "<Air_bPIntkVUsFinalDef>"
  BS_Result/4 -> ToWs_Result_Bus_Sig4/1  "<Air_bPIntkVUsProvDef>"
  BS_Result/5 -> ToWs_Result_Bus_Sig5/1  "<Air_bPhysRngPIntkVUsFinalDef>"
  BS_Result/6 -> ToWs_Result_Bus_Sig6/1  "<Air_bPhysRngPIntkVUsProvDef>"
  BS_Result/7 -> ToWs_Result_Bus_Sig7/1  "<Air_bPlsPIntkVUsFinalDef>"
  BS_Result/8 -> ToWs_Result_Bus_Sig8/1  "<Air_bPlsPIntkVUsProvDef>"
  BS_Result/9 -> ToWs_Result_Bus_Sig9/1  "<Air_bSRCPIntkVUsMaxDeb_DSM>"
  BS_Result/10 -> ToWs_Result_Bus_Sig10/1  "<Air_bSRCPIntkVUsMinDeb_DSM>"
  BS_Result/11 -> ToWs_Result_Bus_Sig11/1  "<Air_bPhysRngPIntkVUsHiDeb_DSM>"
  BS_Result/12 -> ToWs_Result_Bus_Sig12/1  "<Air_bPhysRngPIntkVUsLoDeb_DSM>"
  BS_Result/13 -> ToWs_Result_Bus_Sig13/1  "<Air_bPlsPIntkVUsMaxDeb_DSM>"
  BS_Result/14 -> ToWs_Result_Bus_Sig14/1  "<Air_bPlsPIntkVUsMinDeb_DSM>"
  specifyOutputs/1(result) -> result/1

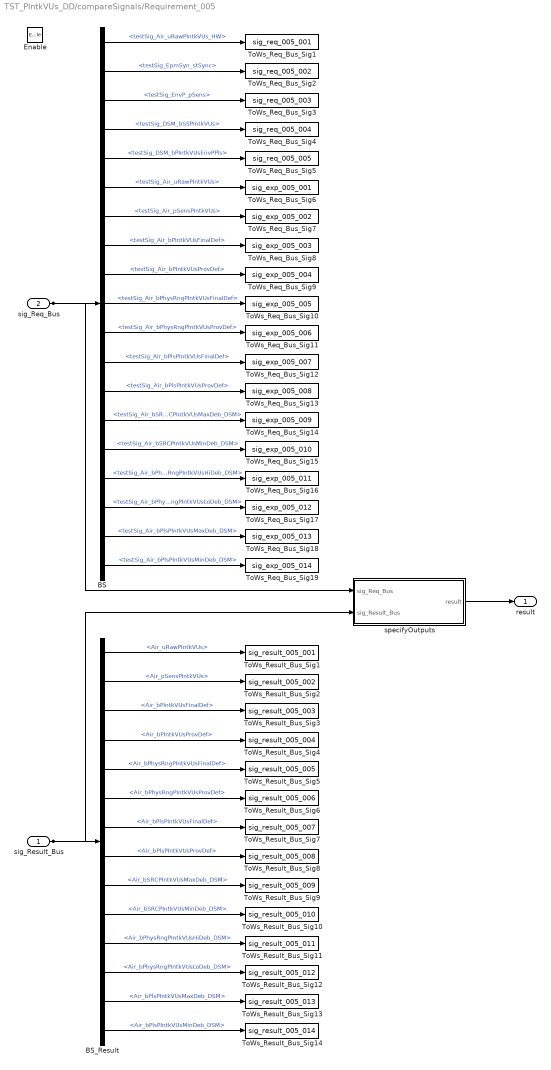
== system TST_PIntkVUs_DD/compareSignals/Requirement_005 ==
  sig_Result_Bus : Inport
  sig_Req_Bus : Inport  Port=2
  Enable : EnablePort
  BS : BusSelector  OutputSignals=testSig_Air_uRawPIntkVUs_HW,testSig_EpmSyn_stSync,testSig_EnvP_pSens,testSig_DSM_bSSPIntkVUs,testSig_DSM_bPIntkVUsEnvPPls,testSig_Air_uRawPIntkVUs,testSig_Air_pSensPIntkVUs,testSig_Air_bPIntkVUsFinalDef,testSig_Air_bPIntkVUsProvDef,testSig_Air_bPhysRngPIntkVUsFinalDef,testSig_Air_bPhysRngPIntkVUsProvDef,testSig_Air_bPlsPIntkVUsFinalDef,testSig_Air_bPlsPIntkVUsProvDef,testSig_Air_bSRCPIntkVUsMaxDeb_DSM,testSig_Air_bSRCPIntkVUsMinDeb_DSM,testSig_Air_bPhysRngPIntkVUsHiDeb_DSM,testSig_Air_bPhysRngPIntkVUsLoDeb_DSM,testSig_Air_bPlsPIntkVUsMaxDeb_DSM,testSig_Air_bPlsPIntkVUsMinDeb_DSM
  BS_Result : BusSelector  OutputSignals=Air_uRawPIntkVUs,Air_pSensPIntkVUs,Air_bPIntkVUsFinalDef,Air_bPIntkVUsProvDef,Air_bPhysRngPIntkVUsFinalDef,Air_bPhysRngPIntkVUsProvDef,Air_bPlsPIntkVUsFinalDef,Air_bPlsPIntkVUsProvDef,Air_bSRCPIntkVUsMaxDeb_DSM,Air_bSRCPIntkVUsMinDeb_DSM,Air_bPhysRngPIntkVUsHiDeb_DSM,Air_bPhysRngPIntkVUsLoDeb_DSM,Air_bPlsPIntkVUsMaxDeb_DSM,Air_bPlsPIntkVUsMinDeb_DSM
  ToWs_Req_Bus_Sig1 : ToWorkspace  VariableName=sig_req_005_001  SaveFormat=Structure With Time
  ToWs_Req_Bus_Sig10 : ToWorkspace  VariableName=sig_exp_005_005  SaveFormat=Structure With Time
  ToWs_Req_Bus_Sig11 : ToWorkspace  VariableName=sig_exp_005_006  SaveFormat=Structure With Time
  ToWs_Req_Bus_Sig12 : ToWorkspace  VariableName=sig_exp_005_007  SaveFormat=Structure With Time
  ToWs_Req_Bus_Sig13 : ToWorkspace  VariableName=sig_exp_005_008  SaveFormat=Structure With Time
  ToWs_Req_Bus_Sig14 : ToWorkspace  VariableName=sig_exp_005_009  SaveFormat=Structure With Time
  ToWs_Req_Bus_Sig15 : ToWorkspace  VariableName=sig_exp_005_010  SaveFormat=Structure With Time
  ToWs_Req_Bus_Sig16 : ToWorkspace  VariableName=sig_exp_005_011  SaveFormat=Structure With Time
  ToWs_Req_Bus_Sig17 : ToWorkspace  VariableName=sig_exp_005_012  SaveFormat=Structure With Time
  ToWs_Req_Bus_Sig18 : ToWorkspace  VariableName=sig_exp_005_013  SaveFormat=Structure With Time
  ToWs_Req_Bus_Sig19 : ToWorkspace  VariableName=sig_exp_005_014  SaveFormat=Structure With Time
  ToWs_Req_Bus_Sig2 : ToWorkspace  VariableName=sig_req_005_002  SaveFormat=Structure With Time
  ToWs_Req_Bus_Sig3 : ToWorkspace  VariableName=sig_req_005_003  SaveFormat=Structure With Time
  ToWs_Req_Bus_Sig4 : ToWorkspace  VariableName=sig_req_005_004  SaveFormat=Structure With Time
  ToWs_Req_Bus_Sig5 : ToWorkspace  VariableName=sig_req_005_005  SaveFormat=Structure With Time
  ToWs_Req_Bus_Sig6 : ToWorkspace  VariableName=sig_exp_005_001  SaveFormat=Structure With Time
  ToWs_Req_Bus_Sig7 : ToWorkspace  VariableName=sig_exp_005_002  SaveFormat=Structure With Time
  ToWs_Req_Bus_Sig8 : ToWorkspace  VariableName=sig_exp_005_003  SaveFormat=Structure With Time
  ToWs_Req_Bus_Sig9 : ToWorkspace  VariableName=sig_exp_005_004  SaveFormat=Structure With Time
  ToWs_Result_Bus_Sig1 : ToWorkspace  VariableName=sig_result_005_001  SaveFormat=Structure With Time
  ToWs_Result_Bus_Sig10 : ToWorkspace  VariableName=sig_result_005_010  SaveFormat=Structure With Time
  ToWs_Result_Bus_Sig11 : ToWorkspace  VariableName=sig_result_005_011  SaveFormat=Structure With Time
  ToWs_Result_Bus_Sig12 : ToWorkspace  VariableName=sig_result_005_012  SaveFormat=Structure With Time
  ToWs_Result_Bus_Sig13 : ToWorkspace  VariableName=sig_result_005_013  SaveFormat=Structure With Time
  ToWs_Result_Bus_Sig14 : ToWorkspace  VariableName=sig_result_005_014  SaveFormat=Structure With Time
  ToWs_Result_Bus_Sig2 : ToWorkspace  VariableName=sig_result_005_002  SaveFormat=Structure With Time
  ToWs_Result_Bus_Sig3 : ToWorkspace  VariableName=sig_result_005_003  SaveFormat=Structure With Time
  ToWs_Result_Bus_Sig4 : ToWorkspace  VariableName=sig_result_005_004  SaveFormat=Structure With Time
  ToWs_Result_Bus_Sig5 : ToWorkspace  VariableName=sig_result_005_005  SaveFormat=Structure With Time
  ToWs_Result_Bus_Sig6 : ToWorkspace  VariableName=sig_result_005_006  SaveFormat=Structure With Time
  ToWs_Result_Bus_Sig7 : ToWorkspace  VariableName=sig_result_005_007  SaveFormat=Structure With Time
  ToWs_Result_Bus_Sig8 : ToWorkspace  VariableName=sig_result_005_008  SaveFormat=Structure With Time
  ToWs_Result_Bus_Sig9 : ToWorkspace  VariableName=sig_result_005_009  SaveFormat=Structure With Time
  specifyOutputs : Subsystem
  result : Outport
  wires:
  sig_Req_Bus/1 -> BS/1, specifyOutputs/1(sig_Req_Bus)
  BS/1 -> ToWs_Req_Bus_Sig1/1  "<testSig_Air_uRawPIntkVUs_HW>"
  BS/2 -> ToWs_Req_Bus_Sig2/1  "<testSig_EpmSyn_stSync>"
  BS/3 -> ToWs_Req_Bus_Sig3/1  "<testSig_EnvP_pSens>"
  BS/4 -> ToWs_Req_Bus_Sig4/1  "<testSig_DSM_bSSPIntkVUs>"
  BS/5 -> ToWs_Req_Bus_Sig5/1  "<testSig_DSM_bPIntkVUsEnvPPls>"
  BS/6 -> ToWs_Req_Bus_Sig6/1  "<testSig_Air_uRawPIntkVUs>"
  BS/7 -> ToWs_Req_Bus_Sig7/1  "<testSig_Air_pSensPIntkVUs>"
  BS/8 -> ToWs_Req_Bus_Sig8/1  "<testSig_Air_bPIntkVUsFinalDef>"
  BS/9 -> ToWs_Req_Bus_Sig9/1  "<testSig_Air_bPIntkVUsProvDef>"
  BS/10 -> ToWs_Req_Bus_Sig10/1  "<testSig_Air_bPhysRngPIntkVUsFinalDef>"
  BS/11 -> ToWs_Req_Bus_Sig11/1  "<testSig_Air_bPhysRngPIntkVUsProvDef>"
  BS/12 -> ToWs_Req_Bus_Sig12/1  "<testSig_Air_bPlsPIntkVUsFinalDef>"
  BS/13 -> ToWs_Req_Bus_Sig13/1  "<testSig_Air_bPlsPIntkVUsProvDef>"
  BS/14 -> ToWs_Req_Bus_Sig14/1  "<testSig_Air_bSRCPIntkVUsMaxDeb_DSM>"
  BS/15 -> ToWs_Req_Bus_Sig15/1  "<testSig_Air_bSRCPIntkVUsMinDeb_DSM>"
  BS/16 -> ToWs_Req_Bus_Sig16/1  "<testSig_Air_bPhysRngPIntkVUsHiDeb_DSM>"
  BS/17 -> ToWs_Req_Bus_Sig17/1  "<testSig_Air_bPhysRngPIntkVUsLoDeb_DSM>"
  BS/18 -> ToWs_Req_Bus_Sig18/1  "<testSig_Air_bPlsPIntkVUsMaxDeb_DSM>"
  BS/19 -> ToWs_Req_Bus_Sig19/1  "<testSig_Air_bPlsPIntkVUsMinDeb_DSM>"
  sig_Result_Bus/1 -> BS_Result/1, specifyOutputs/2(sig_Result_Bus)
  BS_Result/1 -> ToWs_Result_Bus_Sig1/1  "<Air_uRawPIntkVUs>"
  BS_Result/2 -> ToWs_Result_Bus_Sig2/1  "<Air_pSensPIntkVUs>"
  BS_Result/3 -> ToWs_Result_Bus_Sig3/1  "<Air_bPIntkVUsFinalDef>"
  BS_Result/4 -> ToWs_Result_Bus_Sig4/1  "<Air_bPIntkVUsProvDef>"
  BS_Result/5 -> ToWs_Result_Bus_Sig5/1  "<Air_bPhysRngPIntkVUsFinalDef>"
  BS_Result/6 -> ToWs_Result_Bus_Sig6/1  "<Air_bPhysRngPIntkVUsProvDef>"
  BS_Result/7 -> ToWs_Result_Bus_Sig7/1  "<Air_bPlsPIntkVUsFinalDef>"
  BS_Result/8 -> ToWs_Result_Bus_Sig8/1  "<Air_bPlsPIntkVUsProvDef>"
  BS_Result/9 -> ToWs_Result_Bus_Sig9/1  "<Air_bSRCPIntkVUsMaxDeb_DSM>"
  BS_Result/10 -> ToWs_Result_Bus_Sig10/1  "<Air_bSRCPIntkVUsMinDeb_DSM>"
  BS_Result/11 -> ToWs_Result_Bus_Sig11/1  "<Air_bPhysRngPIntkVUsHiDeb_DSM>"
  BS_Result/12 -> ToWs_Result_Bus_Sig12/1  "<Air_bPhysRngPIntkVUsLoDeb_DSM>"
  BS_Result/13 -> ToWs_Result_Bus_Sig13/1  "<Air_bPlsPIntkVUsMaxDeb_DSM>"
  BS_Result/14 -> ToWs_Result_Bus_Sig14/1  "<Air_bPlsPIntkVUsMinDeb_DSM>"
  specifyOutputs/1(result) -> result/1
